simulink model "single_phase_half_wave_controllable_rectification"  (R2023b)
settings: Solver=VariableStepAuto  StartTime=0.0  StopTime=0.1  MaxStep=1e-4  RelTol=1e-3
libraries: spsSeriesRLCBranchLib x2, spsMultimeterLib x1, spsThyristorLib x1, spsACVoltageSourceLib x1, spsMeanLib x1, spsRMSLib x1, sps_lib x1
settings Model: Creator=LuvB4  LastModifiedBy=LuvB4

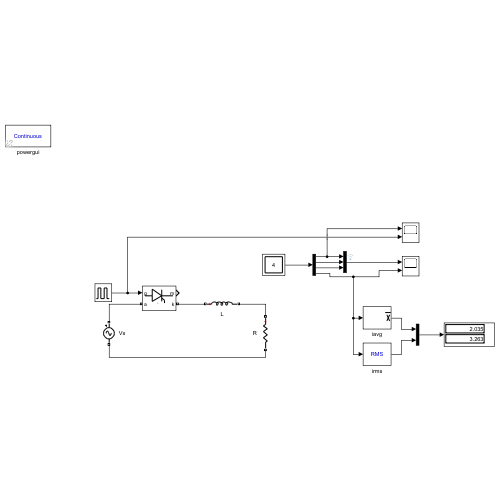
[thumbnail: Simulink's stored preview of the top-level diagram]
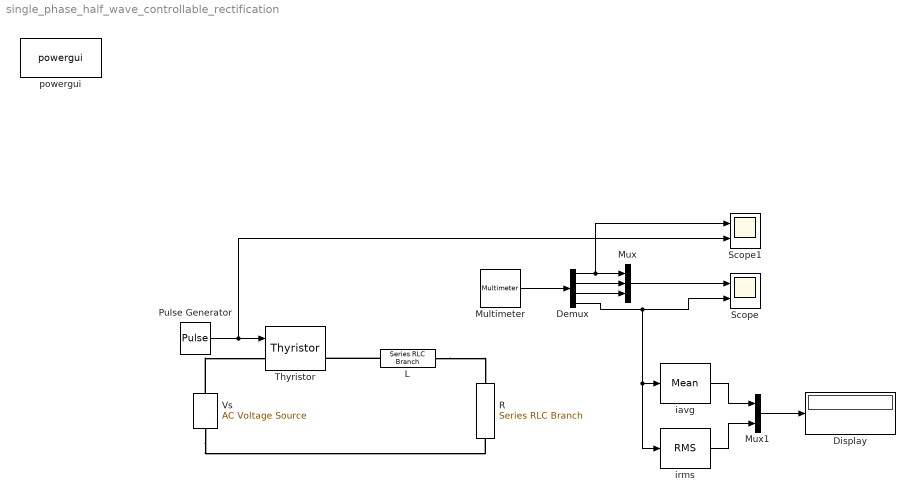
== system single_phase_half_wave_controllable_rectification ==
  Demux : Demux
  Display : Display
  L : spsSeriesRLCBranchLib/Series RLC Branch  LConnTagsString=__new0  RConnTagsString=__new0  BranchType=L  Resistance=10  Inductance=48e-3  SetiL0=off  InitialCurrent=0  Capacitance=1e-6  Setx0=off  InitialVoltage=0  Measurements=Branch voltage
  Multimeter : spsMultimeterLib/Multimeter  L=4  sel=[3 2 1 4]  yselected={}  Gain=[1 1 1 1]  OutputType=Complex  PlotAtSimulationStop=off  PhasorSimulation=off
  Mux : Mux  Inputs=3
  Mux1 : Mux  Inputs=2
  Pulse Generator : DiscretePulseGenerator  PulseType=Time based  Period=1/50  PulseWidth=5  PhaseDelay=(45/360)*(1/50)
  R : spsSeriesRLCBranchLib/Series RLC Branch  LConnTagsString=__new0  RConnTagsString=__new0  BranchType=R  Resistance=20  Inductance=1e-3  SetiL0=off  InitialCurrent=0  Capacitance=1e-6  Setx0=off  InitialVoltage=0  Measurements=Branch voltage and current
  Scope : Scope  NumInputPorts=2
  Scope1 : Scope  NumInputPorts=2
  Thyristor : spsThyristorLib/Thyristor  Ron=0.001  Lon=0  Vf=0  IC=0  Rs=0  Cs=0  Measurements=on
  Vs : spsACVoltageSourceLib/AC Voltage Source  Amplitude=120*sqrt(2)  Phase=0  Frequency=50  SampleTime=0  Measurements=Voltage  BusType=swing  Pref=10e3  Qref=0  Qmin=-inf  Qmax=+inf
  iavg : spsMeanLib/Mean  Freq=50  Vinit=0  Ts=0
  irms : spsRMSLib/RMS  TrueRMS=on  Freq=50  RMSInit=0  Ts=0
  powergui : sps_lib/powergui  Priority=1  SimulationMode=Continuous  SampleTime=50e-6  frequency=60  Iterations=50  frequencyindice=50  Pbase=100e6  ErrMax=1e-4  UnitsV=kV  UnitsW=MW  buscounter=0  FunctionMessages=off  echomessages=off  EnableUseOfTLC=off  CurrentSourceSwitches=off  DisableSnubberDevices=off  DisableRonSwitches=off  DisableVfSwitches=off  DisplayEquations=off  AutomaticDiscreteSolvers=off  SolverType=Tustin/Backward Euler (TBE)  Interpol=off  ExternalGateDelay=off  methode=off  Ts=100  x0status=blocks  SPID=on  SwTol=0  HookPort=off  NonlinearTolerance=1e-4  nMaxIteration=100  ContinueOnMaxIteration=off  RestoreLinks=warning  ResistiveCurrentMeasurement=off  Frange=[0:2:500]  Ylog=off  Xlog=on  ShowGrid=off  save=off  variable=ZData  structure=0  ZoomFFT=off  StartTime=0.0  cycles=1  DisplayStyle=1  fundamental=60  FreqAxis=off  MaxFrequency=1000  frequencyindicesteady=1  RmsSteady=1  display=off
  wires:
  Multimeter/1 -> Demux/1
  Mux/1 -> Scope/1
  Demux/1 -> Scope1/1, Mux/1
  Demux/2 -> Mux/2
  Demux/3 -> Mux/3
  Demux/4 -> irms/1, iavg/1, Scope/2
  Pulse Generator/1 -> Scope1/2, Thyristor/1
  iavg/1 -> Mux1/1
  irms/1 -> Mux1/2
  Mux1/1 -> Display/1
  connections:
  Vs/RConn1 -- Thyristor/LConn1
  Vs/LConn1 -- R/RConn1
  L/LConn1 -- Thyristor/RConn1
  L/RConn1 -- R/LConn1
